simulink model "doc_sawtooth_mod"  (R2014a)
settings: Solver=VariableStepDiscrete  StartTime=0.0  StopTime=10.0  RelTol=1e-3
libraries: commanapbnd3 x2
settings Model: Creator=The MathWorks Inc.
settings DataIOCC: SignalLoggingSaveFormat=ModelDataLogs
settings OptimizationCC: ExpressionDepthLimit=2147483647
settings DebuggingCC: UnderspecifiedInitializationDetection=Classic  FcnCallInpInsideContextMsg=EnableAllAsWarning  StateNameClashWarn=warning

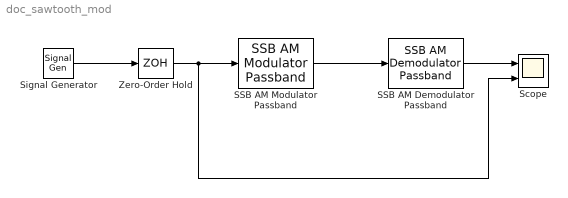
== system doc_sawtooth_mod ==
  SSB AM Demodulator Passband : commanapbnd3/SSB AM Demodulator Passband  Fc=25  Ph=0  method=Butterworth  n=2  cf=30  Rp=0.1  Rs=50
  SSB AM Modulator Passband : commanapbnd3/SSB AM Modulator Passband  Fc=25  Ph=0  Sd=Upper  Ho=200
  Scope : Scope  NumInputPorts=2
      settings: YMin=-5~-5  YMax=5~5
  Signal Generator : SignalGenerator  WaveForm=sawtooth  Amplitude=4  Frequency=.3
  Zero-Order Hold : ZeroOrderHold  SampleTime=.01
  wires:
  Signal Generator/1 -> Zero-Order Hold/1
  Zero-Order Hold/1 -> SSB AM Modulator Passband/1, Scope/2
  SSB AM Modulator Passband/1 -> SSB AM Demodulator Passband/1
  SSB AM Demodulator Passband/1 -> Scope/1
